simulink model "BBB_with_I2CPWMboard"  (R2020b)
settings: Solver=FixedStepAuto  StartTime=0.0  StopTime=inf  RelTol=1e-3  EnableMultiTasking=on
libraries: bbblueCommlib x3
settings Model: ExtModeTrigDuration=100  Creator=ONLY-GOD  LastModifiedBy=ONLY-GOD
settings SolverCC: PositivePriorityOrder=on
settings OptimizationCC: EnhancedBackFolding=on  PassReuseOutputArgsAs=Individual arguments  ZeroExternalMemoryAtStartup=off  ZeroInternalMemoryAtStartup=off  MaxStackSize=64  OptimizeBlockOrder=speed  DifferentSizesBufferReuse=on  OptimizationCustomize=off  EfficientTunableParamExpr=on
settings DebuggingCC: ParameterTunabilityLossMsg=error
settings HardwareCC: ProdBitPerPointer=32  ProdBitPerSizeT=32  ProdBitPerPtrDiffT=32  ProdLargestAtomicInteger=Long  ProdLargestAtomicFloat=Double  ProdWordSize=32  ProdHWDeviceType=ARM Compatible->ARM Cortex
settings SFSimCC: MATLABDynamicMemAlloc=off
settings RTWCC: Description=Embedded Coder  SystemTargetFile=ert.tlc  HardwareBoard=BeagleBone Blue  TLCOptions="-aInlineSetEventsForThisBaseRateFcn=TLC_FALSE -aSuppressMultiTaskScheduler=TLC_FALSE  -aRateBasedStepFcn=0"  TemplateMakefile=ert_default_tmf  GenerateReport=on  Toolchain=GNU GCC BeagleBone Blue  IncludeHyperlinkInReport=on  LaunchReport=on  GenerateTraceInfo=on  GenerateTraceReport=on  GenerateTraceReportSl=on  GenerateTraceReportSf=on  GenerateTraceReportEml=on
settings CodeAppCC: ForceParamTrailComments=on  IgnoreCustomStorageClasses=off  OperatorAnnotations=on  SimulinkDataObjDesc=on  SFDataObjDesc=on  InsertBlockDesc=on
settings ERTTargetCC: SupportVariableSizeSignals=on

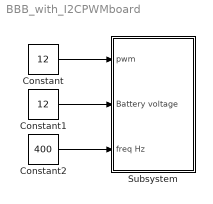
== system BBB_with_I2CPWMboard ==
  Constant : Constant  Value=12
  Constant1 : Constant  Value=12
  Constant2 : Constant  Value=400
  Subsystem : Subsystem
  wires:
  Constant1/1 -> Subsystem/2(Battery voltage)
  Constant/1 -> Subsystem/1(pwm)
  Constant2/1 -> Subsystem/3(freq Hz)

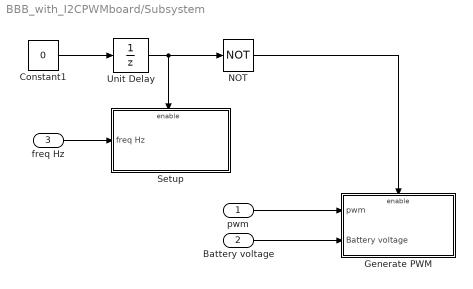
== system BBB_with_I2CPWMboard/Subsystem ==
  pwm : Inport
  Battery voltage : Inport  Port=2
  freq Hz : Inport  Port=3
  Constant1 : Constant  Value=0
  Generate PWM : Subsystem
  NOT : Logic  Operator=NOT  IconShape=distinctive  AllPortsSameDT=off  OutDataTypeStr=boolean
  Setup : Subsystem
  Unit Delay : UnitDelay  InitialCondition=1  SampleTime=-1  HasFrameUpgradeWarning=on
  wires:
  Battery voltage/1 -> Generate PWM/2(Battery voltage)
  Constant1/1 -> Unit Delay/1
  NOT/1 -> Generate PWM/Enable
  pwm/1 -> Generate PWM/1(pwm)
  freq Hz/1 -> Setup/1(freq Hz)
  Unit Delay/1 -> NOT/1, Setup/Enable

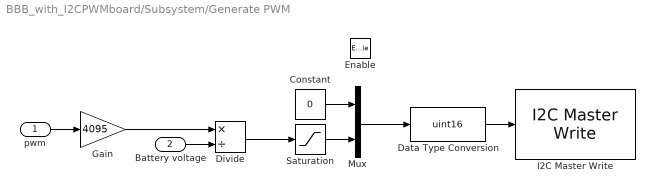
== system BBB_with_I2CPWMboard/Subsystem/Generate PWM ==
  pwm : Inport
  Battery voltage : Inport  Port=2
  Enable : EnablePort
  Constant : Constant  Value=0
  Data Type Conversion : DataTypeConversion  OutDataTypeStr=uint16
  Divide : Product  Inputs=*/
  Gain : Gain  Gain=4095
  I2C Master Write : bbblueCommlib/I2C Master Write  I2CModule=1  Mode=Master  SlaveAddress="uint8(hex2dec(\"40\"))"  SlaveByteOrder=LittleEndian  Direction=Transmitter  RegisterAddressMode=on  RegisterAddress=uint8(6)  SlaveDataType=uint8  DataLength=1  NoAck=off  RepeatedStart=off  OutputStatus=off
      settings: SourceProductBaseCode=SC_BEAGLEBONE_BLUE
  Mux : Mux  Inputs=2
  Saturation : Saturate  UpperLimit=4095  LowerLimit=0
  wires:
  Mux/1 -> Data Type Conversion/1
  pwm/1 -> Gain/1
  Battery voltage/1 -> Divide/2
  Data Type Conversion/1 -> I2C Master Write/1
  Divide/1 -> Saturation/1
  Saturation/1 -> Mux/2
  Constant/1 -> Mux/1
  Gain/1 -> Divide/1

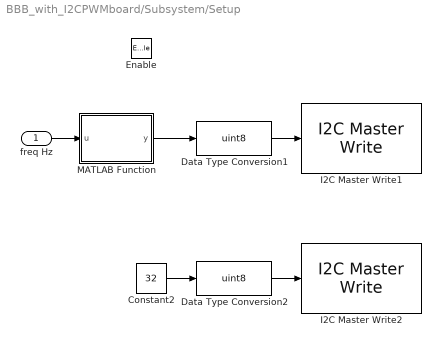
== system BBB_with_I2CPWMboard/Subsystem/Setup ==
  freq Hz : Inport
  Enable : EnablePort
  Constant2 : Constant  Value=32
  Data Type Conversion1 : DataTypeConversion  OutDataTypeStr=uint8
  Data Type Conversion2 : DataTypeConversion  OutDataTypeStr=uint8
  I2C Master Write1 : bbblueCommlib/I2C Master Write  I2CModule=1  Mode=Master  SlaveAddress="uint8(hex2dec(\"40\"))"  SlaveByteOrder=LittleEndian  Direction=Transmitter  RegisterAddressMode=on  RegisterAddress="uint8(hex2dec(\"FE\"))"  SlaveDataType=uint8  DataLength=1  NoAck=off  RepeatedStart=off  OutputStatus=off
      settings: SourceProductBaseCode=SC_BEAGLEBONE_BLUE
  I2C Master Write2 : bbblueCommlib/I2C Master Write  I2CModule=1  Mode=Master  SlaveAddress="uint8(hex2dec(\"40\"))"  SlaveByteOrder=LittleEndian  Direction=Transmitter  RegisterAddressMode=on  RegisterAddress="uint8(hex2dec(\"00\"))"  SlaveDataType=uint8  DataLength=1  NoAck=off  RepeatedStart=off  OutputStatus=off
      settings: SourceProductBaseCode=SC_BEAGLEBONE_BLUE
  MATLAB Function : MATLAB Function  TreatAsAtomicUnit=on
  wires:
  Data Type Conversion2/1 -> I2C Master Write2/1
  Constant2/1 -> Data Type Conversion2/1
  Data Type Conversion1/1 -> I2C Master Write1/1
  MATLAB Function/1(y) -> Data Type Conversion1/1
  freq Hz/1 -> MATLAB Function/1(u)

== matlab function BBB_with_I2CPWMboard/Subsystem/Setup/MATLAB Function ==
  data: u input; y output
function y = fcn(u)

y = fix(25e6/4096/u)-1;
